simulink model "visualization_of_quad"  (R2015a)
settings: Solver=ode45  StartTime=0.0  StopTime=inf  RelTol=1e-3
values from neighbouring files (symbols this model uses):
  Beq = 0.2    [Parametres.m]
  Jeq = 0.005    [Parametres.m]
  Kb = 12    [Parametres.m]
  Kt = 12    [Parametres.m]
  Nl = 100    [Parametres.m]
  Nm = 200    [Parametres.m]
  Ra = 1100    [Parametres.m]
undefined symbols (not defined in the file or in its folder): sigbuilder_block
libraries: mblibv1 x34, simulink x5
settings Model: Creator=clien  LastModifiedBy=user
settings DataIOCC: SignalLoggingSaveFormat=ModelDataLogs
settings OptimizationCC: ExpressionDepthLimit=2147483647
settings DebuggingCC: UnderspecifiedInitializationDetection=Classic  MergeDetectMultiDrivingBlocksExec=none  SolverPrmCheckMsg=warning  FcnCallInpInsideContextMsg=UseLocalSettings  StateNameClashWarn=warning
settings GRTTargetCC: CombineOutputUpdateFcns=off  GRTInterface=on
settings SimMechanicsCC: VisOnUpdateDiagram=on  VisDuringSimulation=on  AutoFitVis=TIGHTFIT  LastVizWinPosition=[1 41 1366 627]  CamPosition=[6.82801;6.80801;6.82801;]  CamTarget=[-8.88178e-16;-0.02;-8.88178e-16;]  CamUpVector=[0;1;0;]  CamHeight=1.02417  VisBackgroundColor=[0.9;0.9;0.95;]  DefaultBodyColor=[1;0;0;]

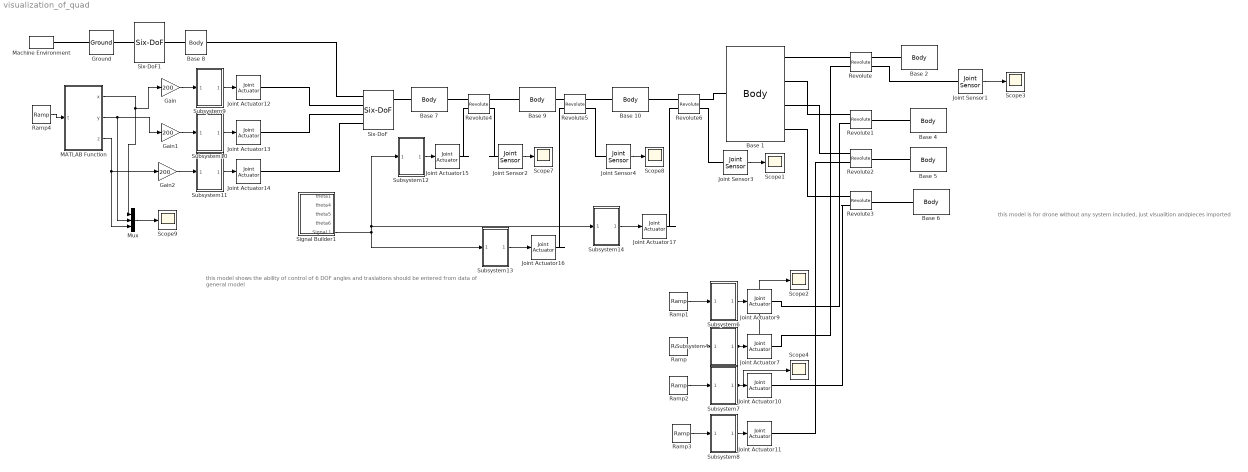
== system visualization_of_quad ==
  note: this model shows the ability of control of 6 DOF angles and traslations should be entered
      | from data of general model
  note: this model is for drone without any system included, just visualition andpieces imported
  Base 1 : mblibv1/Bodies/Body  LConnTagsString=CS1  RConnTagsString=CS5|CS4|CS3|CS2  UpdateFromCAD=off  DialogClass=MechanicalBodyBlock  Mass=.001  MassUnits=kg  InertiaUnits=kg*m^2  Inertia=eye(3)  Shape=Cylinder  ShapeDims=[1 1]  ShapeUnits=m  ShapeUse=false  Density=1  DensityUnits=kg/m^3  DensityUse=false  GraphicsMode=GFXFILE  GraphicsFileName=C:\Users\Oussama\Desktop\str file FINAL\framebody.stl  BodyColorSelMode=COLORPALETTE  BodyColor=[1 0.84314 0]  AttachedToCS=CS1  CG=Left$CG$[0 0 0]$World$CS1$mm$[0 0 0]$Euler X-Y-Z$deg$WORLD$false$none  WorkingFrames=Right$CS5$[0 30 -300]$Adjoining$CS1$mm$[0 0 0]$Euler X-Y-Z$deg$WORLD$true$none#Right$CS4$[0 30 300]$Adjoining$CS1$mm$[0 0 0]$Euler X-Y-Z$deg$WORLD$true$none#Right$CS3$[300 30 0]$Adjoining$CS1$mm$[0 0 0]$Euler X-Y-Z$deg$WORLD$true$none#Left$CS1$[0 0 0]$Adjoining$Adjoining$mm$[0 0 0]$Euler X-Y-Z$deg$WORLD$true$none#Right$CS2$[-300 30 0]$Adjoining$CS1$mm$[0 0 0]$Euler X-Y-Z$deg$WORLD$true$none  CGPos=[0 0 0]  CGRot=[0 0 0]  CS0Pos=[]  CS0Rot=[]  CS1Pos=[0 0 0]  CS1Rot=[0 0 0]  CS2Pos=[-300 30 0]  CS2Rot=[0 0 0]  CS3Pos=[300 30 0]  CS3Rot=[0 0 0]  CS4Pos=[0 30 300]  CS4Rot=[0 0 0]  CS5Pos=[0 30 -300]  CS5Rot=[0 0 0]  CS6Pos=[]  CS6Rot=[]  CS7Pos=[]  CS7Rot=[]  CS8Pos=[]  CS8Rot=[]  CS9Pos=[]  CS9Rot=[]  CS10Pos=[]  CS10Rot=[]  CS11Pos=[]  CS11Rot=[]  CS12Pos=[]  CS12Rot=[]  CS13Pos=[]  CS13Rot=[]  CS14Pos=[]  CS14Rot=[]  CS15Pos=[]  CS15Rot=[]  CS16Pos=[]  CS16Rot=[]  CS17Pos=[]  CS17Rot=[]  CS18Pos=[]  CS18Rot=[]  CS19Pos=[]  CS19Rot=[]  CS20Pos=[]  CS20Rot=[]
  Base 10 : mblibv1/Bodies/Body  LConnTagsString=CS1  RConnTagsString=CS2  UpdateFromCAD=off  DialogClass=MechanicalBodyBlock  Mass=0.00001  MassUnits=kg  InertiaUnits=kg*m^2  Inertia=eye(3)  Shape=Cylinder  ShapeDims=[1 1]  ShapeUnits=m  ShapeUse=false  Density=1  DensityUnits=kg/m^3  DensityUse=false  GraphicsMode=MACHINE_DEFAULT  GraphicsFileName=C:\Users\Oussama\Desktop\str file FINAL\framebody.stl  BodyColorSelMode=COLORPALETTE  BodyColor=[0 0 0]  AttachedToCS=CS1  CG=Left$CG$[0 0 0]$World$CS1$mm$[0 0 0]$Euler X-Y-Z$deg$WORLD$false$none  WorkingFrames=Left$CS1$[0 0 0]$Adjoining$Adjoining$mm$[0 0 0]$Euler X-Y-Z$deg$WORLD$true$none#Right$CS2$[0 0 0]$World$CS1$mm$[0 0 0]$Euler X-Y-Z$deg$WORLD$true$none  CGPos=[0 0 0]  CGRot=[0 0 0]  CS0Pos=[]  CS0Rot=[]  CS1Pos=[0 0 0]  CS1Rot=[0 0 0]  CS2Pos=[0 0 0]  CS2Rot=[0 0 0]  CS3Pos=[]  CS3Rot=[]  CS4Pos=[]  CS4Rot=[]  CS5Pos=[]  CS5Rot=[]  CS6Pos=[]  CS6Rot=[]  CS7Pos=[]  CS7Rot=[]  CS8Pos=[]  CS8Rot=[]  CS9Pos=[]  CS9Rot=[]  CS10Pos=[]  CS10Rot=[]  CS11Pos=[]  CS11Rot=[]  CS12Pos=[]  CS12Rot=[]  CS13Pos=[]  CS13Rot=[]  CS14Pos=[]  CS14Rot=[]  CS15Pos=[]  CS15Rot=[]  CS16Pos=[]  CS16Rot=[]  CS17Pos=[]  CS17Rot=[]  CS18Pos=[]  CS18Rot=[]  CS19Pos=[]  CS19Rot=[]  CS20Pos=[]  CS20Rot=[]
  Base 2 : mblibv1/Bodies/Body  LConnTagsString=CS1  RConnTagsString=CS2  UpdateFromCAD=off  DialogClass=MechanicalBodyBlock  Mass=0.000001  MassUnits=kg  InertiaUnits=kg*m^2  Inertia=eye(3)  Shape=Cylinder  ShapeDims=[1 1]  ShapeUnits=m  ShapeUse=false  Density=1  DensityUnits=kg/m^3  DensityUse=false  GraphicsMode=GFXFILE  GraphicsFileName=C:\Users\Oussama\Desktop\str file FINAL\proplers.stl  BodyColorSelMode=COLORPALETTE  BodyColor=[1 0 0]  AttachedToCS=CS1  CG=Left$CG$[0 0 0]$World$CS1$mm$[0 0 0]$Euler X-Y-Z$deg$WORLD$false$none  WorkingFrames=Left$CS1$[0 0 0]$Adjoining$Adjoining$mm$[0 0 0]$Euler X-Y-Z$deg$WORLD$true$none#Right$CS2$[0 0 0]$World$CS1$mm$[0 0 0]$Euler X-Y-Z$deg$WORLD$true$none  CGPos=[0 0 0]  CGRot=[0 0 0]  CS0Pos=[]  CS0Rot=[]  CS1Pos=[0 0 0]  CS1Rot=[0 0 0]  CS2Pos=[0 0 0]  CS2Rot=[0 0 0]  CS3Pos=[]  CS3Rot=[]  CS4Pos=[]  CS4Rot=[]  CS5Pos=[]  CS5Rot=[]  CS6Pos=[]  CS6Rot=[]  CS7Pos=[]  CS7Rot=[]  CS8Pos=[]  CS8Rot=[]  CS9Pos=[]  CS9Rot=[]  CS10Pos=[]  CS10Rot=[]  CS11Pos=[]  CS11Rot=[]  CS12Pos=[]  CS12Rot=[]  CS13Pos=[]  CS13Rot=[]  CS14Pos=[]  CS14Rot=[]  CS15Pos=[]  CS15Rot=[]  CS16Pos=[]  CS16Rot=[]  CS17Pos=[]  CS17Rot=[]  CS18Pos=[]  CS18Rot=[]  CS19Pos=[]  CS19Rot=[]  CS20Pos=[]  CS20Rot=[]
  Base 4 : mblibv1/Bodies/Body  LConnTagsString=CS1  RConnTagsString=CS2  UpdateFromCAD=off  DialogClass=MechanicalBodyBlock  Mass=0.000001  MassUnits=kg  InertiaUnits=kg*m^2  Inertia=eye(3)  Shape=Cylinder  ShapeDims=[1 1]  ShapeUnits=m  ShapeUse=false  Density=1  DensityUnits=kg/m^3  DensityUse=false  GraphicsMode=GFXFILE  GraphicsFileName=C:\Users\Oussama\Desktop\str file FINAL\proplers.stl  BodyColorSelMode=COLORPALETTE  BodyColor=[1 0 1]  AttachedToCS=CS1  CG=Left$CG$[0 0 0]$World$CS1$mm$[0 0 0]$Euler X-Y-Z$deg$WORLD$false$none  WorkingFrames=Left$CS1$[0 0 0]$Adjoining$Adjoining$mm$[0 0 0]$Euler X-Y-Z$deg$WORLD$true$none#Right$CS2$[0 0 0]$World$CS1$mm$[0 0 0]$Euler X-Y-Z$deg$WORLD$true$none  CGPos=[0 0 0]  CGRot=[0 0 0]  CS0Pos=[]  CS0Rot=[]  CS1Pos=[0 0 0]  CS1Rot=[0 0 0]  CS2Pos=[0 0 0]  CS2Rot=[0 0 0]  CS3Pos=[]  CS3Rot=[]  CS4Pos=[]  CS4Rot=[]  CS5Pos=[]  CS5Rot=[]  CS6Pos=[]  CS6Rot=[]  CS7Pos=[]  CS7Rot=[]  CS8Pos=[]  CS8Rot=[]  CS9Pos=[]  CS9Rot=[]  CS10Pos=[]  CS10Rot=[]  CS11Pos=[]  CS11Rot=[]  CS12Pos=[]  CS12Rot=[]  CS13Pos=[]  CS13Rot=[]  CS14Pos=[]  CS14Rot=[]  CS15Pos=[]  CS15Rot=[]  CS16Pos=[]  CS16Rot=[]  CS17Pos=[]  CS17Rot=[]  CS18Pos=[]  CS18Rot=[]  CS19Pos=[]  CS19Rot=[]  CS20Pos=[]  CS20Rot=[]
  Base 5 : mblibv1/Bodies/Body  LConnTagsString=CS1  RConnTagsString=CS2  UpdateFromCAD=off  DialogClass=MechanicalBodyBlock  Mass=0.000001  MassUnits=kg  InertiaUnits=kg*m^2  Inertia=eye(3)  Shape=Cylinder  ShapeDims=[1 1]  ShapeUnits=m  ShapeUse=false  Density=1  DensityUnits=kg/m^3  DensityUse=false  GraphicsMode=GFXFILE  GraphicsFileName=C:\Users\Oussama\Desktop\str file FINAL\proplers.stl  BodyColorSelMode=COLORPALETTE  BodyColor=[0 0 1]  AttachedToCS=CS1  CG=Left$CG$[0 0 0]$World$CS1$mm$[0 0 0]$Euler X-Y-Z$deg$WORLD$false$none  WorkingFrames=Left$CS1$[0 0 0]$Adjoining$Adjoining$mm$[0 0 0]$Euler X-Y-Z$deg$WORLD$true$none#Right$CS2$[0 0 0]$World$CS1$mm$[0 0 0]$Euler X-Y-Z$deg$WORLD$true$none  CGPos=[0 0 0]  CGRot=[0 0 0]  CS0Pos=[]  CS0Rot=[]  CS1Pos=[0 0 0]  CS1Rot=[0 0 0]  CS2Pos=[0 0 0]  CS2Rot=[0 0 0]  CS3Pos=[]  CS3Rot=[]  CS4Pos=[]  CS4Rot=[]  CS5Pos=[]  CS5Rot=[]  CS6Pos=[]  CS6Rot=[]  CS7Pos=[]  CS7Rot=[]  CS8Pos=[]  CS8Rot=[]  CS9Pos=[]  CS9Rot=[]  CS10Pos=[]  CS10Rot=[]  CS11Pos=[]  CS11Rot=[]  CS12Pos=[]  CS12Rot=[]  CS13Pos=[]  CS13Rot=[]  CS14Pos=[]  CS14Rot=[]  CS15Pos=[]  CS15Rot=[]  CS16Pos=[]  CS16Rot=[]  CS17Pos=[]  CS17Rot=[]  CS18Pos=[]  CS18Rot=[]  CS19Pos=[]  CS19Rot=[]  CS20Pos=[]  CS20Rot=[]
  Base 6 : mblibv1/Bodies/Body  LConnTagsString=CS1  RConnTagsString=CS2  UpdateFromCAD=off  DialogClass=MechanicalBodyBlock  Mass=0.000001  MassUnits=kg  InertiaUnits=kg*m^2  Inertia=eye(3)  Shape=Cylinder  ShapeDims=[1 1]  ShapeUnits=m  ShapeUse=false  Density=1  DensityUnits=kg/m^3  DensityUse=false  GraphicsMode=GFXFILE  GraphicsFileName=C:\Users\Oussama\Desktop\str file FINAL\proplers.stl  BodyColorSelMode=COLORPALETTE  BodyColor=[0 1 0]  AttachedToCS=CS1  CG=Left$CG$[0 0 0]$World$CS1$mm$[0 0 0]$Euler X-Y-Z$deg$WORLD$false$none  WorkingFrames=Left$CS1$[0 0 0]$Adjoining$Adjoining$mm$[0 0 0]$Euler X-Y-Z$deg$WORLD$true$none#Right$CS2$[0 0 0]$World$CS1$mm$[0 0 0]$Euler X-Y-Z$deg$WORLD$true$none  CGPos=[0 0 0]  CGRot=[0 0 0]  CS0Pos=[]  CS0Rot=[]  CS1Pos=[0 0 0]  CS1Rot=[0 0 0]  CS2Pos=[0 0 0]  CS2Rot=[0 0 0]  CS3Pos=[]  CS3Rot=[]  CS4Pos=[]  CS4Rot=[]  CS5Pos=[]  CS5Rot=[]  CS6Pos=[]  CS6Rot=[]  CS7Pos=[]  CS7Rot=[]  CS8Pos=[]  CS8Rot=[]  CS9Pos=[]  CS9Rot=[]  CS10Pos=[]  CS10Rot=[]  CS11Pos=[]  CS11Rot=[]  CS12Pos=[]  CS12Rot=[]  CS13Pos=[]  CS13Rot=[]  CS14Pos=[]  CS14Rot=[]  CS15Pos=[]  CS15Rot=[]  CS16Pos=[]  CS16Rot=[]  CS17Pos=[]  CS17Rot=[]  CS18Pos=[]  CS18Rot=[]  CS19Pos=[]  CS19Rot=[]  CS20Pos=[]  CS20Rot=[]
  Base 7 : mblibv1/Bodies/Body  LConnTagsString=CS1  RConnTagsString=CS2  UpdateFromCAD=off  DialogClass=MechanicalBodyBlock  Mass=100000  MassUnits=kg  InertiaUnits=kg*m^2  Inertia=1000000*eye(3)  Shape=Cylinder  ShapeDims=[1 1]  ShapeUnits=m  ShapeUse=false  Density=1  DensityUnits=kg/m^3  DensityUse=false  GraphicsMode=MACHINE_DEFAULT  GraphicsFileName=C:\Users\Oussama\Desktop\str file FINAL\framebody.stl  BodyColorSelMode=COLORPALETTE  BodyColor=[0 0 0]  AttachedToCS=CS1  CG=Left$CG$[0 0 0]$World$CS1$mm$[0 0 0]$Euler X-Y-Z$deg$WORLD$false$none  WorkingFrames=Left$CS1$[0 0 0]$Adjoining$Adjoining$mm$[0 0 0]$Euler X-Y-Z$deg$WORLD$true$none#Right$CS2$[0 0 0]$World$CS1$mm$[0 0 0]$Euler X-Y-Z$deg$WORLD$true$none  CGPos=[0 0 0]  CGRot=[0 0 0]  CS0Pos=[]  CS0Rot=[]  CS1Pos=[0 0 0]  CS1Rot=[0 0 0]  CS2Pos=[0 0 0]  CS2Rot=[0 0 0]  CS3Pos=[]  CS3Rot=[]  CS4Pos=[]  CS4Rot=[]  CS5Pos=[]  CS5Rot=[]  CS6Pos=[]  CS6Rot=[]  CS7Pos=[]  CS7Rot=[]  CS8Pos=[]  CS8Rot=[]  CS9Pos=[]  CS9Rot=[]  CS10Pos=[]  CS10Rot=[]  CS11Pos=[]  CS11Rot=[]  CS12Pos=[]  CS12Rot=[]  CS13Pos=[]  CS13Rot=[]  CS14Pos=[]  CS14Rot=[]  CS15Pos=[]  CS15Rot=[]  CS16Pos=[]  CS16Rot=[]  CS17Pos=[]  CS17Rot=[]  CS18Pos=[]  CS18Rot=[]  CS19Pos=[]  CS19Rot=[]  CS20Pos=[]  CS20Rot=[]
  Base 8 : mblibv1/Bodies/Body  LConnTagsString=CS1  RConnTagsString=CS2  UpdateFromCAD=off  DialogClass=MechanicalBodyBlock  Mass=100000000000000000000  MassUnits=kg  InertiaUnits=kg*m^2  Inertia=10000000000000000*eye(3)  Shape=Cylinder  ShapeDims=[1 1]  ShapeUnits=m  ShapeUse=false  Density=1  DensityUnits=kg/m^3  DensityUse=false  GraphicsMode=MACHINE_DEFAULT  GraphicsFileName=C:\Users\Oussama\Desktop\str file FINAL\framebody.stl  BodyColorSelMode=COLORPALETTE  BodyColor=[0 0 0]  AttachedToCS=CS1  CG=Left$CG$[0 0 0]$World$CS1$mm$[0 0 0]$Euler X-Y-Z$deg$WORLD$false$none  WorkingFrames=Left$CS1$[0 0 0]$Adjoining$Adjoining$mm$[0 0 0]$Euler X-Y-Z$deg$WORLD$true$none#Right$CS2$[0 0 0]$World$CS1$mm$[0 0 0]$Euler X-Y-Z$deg$WORLD$true$none  CGPos=[0 0 0]  CGRot=[0 0 0]  CS0Pos=[]  CS0Rot=[]  CS1Pos=[0 0 0]  CS1Rot=[0 0 0]  CS2Pos=[0 0 0]  CS2Rot=[0 0 0]  CS3Pos=[]  CS3Rot=[]  CS4Pos=[]  CS4Rot=[]  CS5Pos=[]  CS5Rot=[]  CS6Pos=[]  CS6Rot=[]  CS7Pos=[]  CS7Rot=[]  CS8Pos=[]  CS8Rot=[]  CS9Pos=[]  CS9Rot=[]  CS10Pos=[]  CS10Rot=[]  CS11Pos=[]  CS11Rot=[]  CS12Pos=[]  CS12Rot=[]  CS13Pos=[]  CS13Rot=[]  CS14Pos=[]  CS14Rot=[]  CS15Pos=[]  CS15Rot=[]  CS16Pos=[]  CS16Rot=[]  CS17Pos=[]  CS17Rot=[]  CS18Pos=[]  CS18Rot=[]  CS19Pos=[]  CS19Rot=[]  CS20Pos=[]  CS20Rot=[]
  Base 9 : mblibv1/Bodies/Body  LConnTagsString=CS1  RConnTagsString=CS2  UpdateFromCAD=off  DialogClass=MechanicalBodyBlock  Mass=0.00001  MassUnits=kg  InertiaUnits=kg*m^2  Inertia=eye(3)  Shape=Cylinder  ShapeDims=[1 1]  ShapeUnits=m  ShapeUse=false  Density=1  DensityUnits=kg/m^3  DensityUse=false  GraphicsMode=MACHINE_DEFAULT  GraphicsFileName=C:\Users\Oussama\Desktop\str file FINAL\framebody.stl  BodyColorSelMode=COLORPALETTE  BodyColor=[0 0 0]  AttachedToCS=CS1  CG=Left$CG$[0 0 0]$World$CS1$mm$[0 0 0]$Euler X-Y-Z$deg$WORLD$false$none  WorkingFrames=Left$CS1$[0 0 0]$Adjoining$Adjoining$mm$[0 0 0]$Euler X-Y-Z$deg$WORLD$true$none#Right$CS2$[0 0 0]$World$CS1$mm$[0 0 0]$Euler X-Y-Z$deg$WORLD$true$none  CGPos=[0 0 0]  CGRot=[0 0 0]  CS0Pos=[]  CS0Rot=[]  CS1Pos=[0 0 0]  CS1Rot=[0 0 0]  CS2Pos=[0 0 0]  CS2Rot=[0 0 0]  CS3Pos=[]  CS3Rot=[]  CS4Pos=[]  CS4Rot=[]  CS5Pos=[]  CS5Rot=[]  CS6Pos=[]  CS6Rot=[]  CS7Pos=[]  CS7Rot=[]  CS8Pos=[]  CS8Rot=[]  CS9Pos=[]  CS9Rot=[]  CS10Pos=[]  CS10Rot=[]  CS11Pos=[]  CS11Rot=[]  CS12Pos=[]  CS12Rot=[]  CS13Pos=[]  CS13Rot=[]  CS14Pos=[]  CS14Rot=[]  CS15Pos=[]  CS15Rot=[]  CS16Pos=[]  CS16Rot=[]  CS17Pos=[]  CS17Rot=[]  CS18Pos=[]  CS18Rot=[]  CS19Pos=[]  CS19Rot=[]  CS20Pos=[]  CS20Rot=[]
  Gain : Gain  Gain=200
  Gain1 : Gain  Gain=200
  Gain2 : Gain  Gain=200
  Ground : mblibv1/Bodies/Ground  UpdateFromCAD=off  LeftPortType=env  RightPortType=workingframe  PhysicalDomain=Mechanical  DialogClass=GroundBlock  CoordPosition=[0 0 0]  CoordPositionUnits=m  StateVectorMgrId=0  MachineId=[1 0]  ShowEnvPort=on  ParameterChecksum=[2469406994, 1823206531, 3009068099, 3398779523]  TopologyChecksum=[157137947, 283279318, 358089753, 4107751040]
  Joint Actuator10 : mblibv1/Sensors &  Actuators/Joint Actuator  UpdateFromCAD=off  PhysicalDomain=Mechanical  PortType=blob  ActuationStyle=Motion  AngleUnits=rev  ArcVelocityUnits=rpm  ArcAccelerationUnits=rad/s^2  CoordPositionUnits=m  VelocityUnits=m/s  AccelerationUnits=m/s^2  ForceUnits=N  TorqueUnits=N*m  ActiveIO=on  Width=3  DialogClass=MechanicalActuatorBlock  Primitive=R1  ReferenceFrame=Absolute (World)
  Joint Actuator11 : mblibv1/Sensors &  Actuators/Joint Actuator  UpdateFromCAD=off  PhysicalDomain=Mechanical  PortType=blob  ActuationStyle=Motion  AngleUnits=rev  ArcVelocityUnits=rad/s  ArcAccelerationUnits=rad/s^2  CoordPositionUnits=m  VelocityUnits=m/s  AccelerationUnits=m/s^2  ForceUnits=N  TorqueUnits=N*m  ActiveIO=on  Width=3  DialogClass=MechanicalActuatorBlock  Primitive=R1  ReferenceFrame=Absolute (World)
  Joint Actuator12 : mblibv1/Sensors &  Actuators/Joint Actuator  UpdateFromCAD=off  PhysicalDomain=Mechanical  PortType=blob  ActuationStyle=Motion  AngleUnits=rev  ArcVelocityUnits=rpm  ArcAccelerationUnits=rad/s^2  CoordPositionUnits=mm  VelocityUnits=m/s  AccelerationUnits=m/s^2  ForceUnits=N  TorqueUnits=N*m  ActiveIO=on  Width=3  DialogClass=MechanicalActuatorBlock  Primitive=P1  ReferenceFrame=Absolute (World)
  Joint Actuator13 : mblibv1/Sensors &  Actuators/Joint Actuator  UpdateFromCAD=off  PhysicalDomain=Mechanical  PortType=blob  ActuationStyle=Motion  AngleUnits=rev  ArcVelocityUnits=rpm  ArcAccelerationUnits=rad/s^2  CoordPositionUnits=mm  VelocityUnits=m/s  AccelerationUnits=m/s^2  ForceUnits=N  TorqueUnits=N*m  ActiveIO=on  Width=3  DialogClass=MechanicalActuatorBlock  Primitive=P3  ReferenceFrame=Absolute (World)
  Joint Actuator14 : mblibv1/Sensors &  Actuators/Joint Actuator  UpdateFromCAD=off  PhysicalDomain=Mechanical  PortType=blob  ActuationStyle=Motion  AngleUnits=rev  ArcVelocityUnits=rpm  ArcAccelerationUnits=rad/s^2  CoordPositionUnits=mm  VelocityUnits=m/s  AccelerationUnits=m/s^2  ForceUnits=N  TorqueUnits=N*m  ActiveIO=on  Width=3  DialogClass=MechanicalActuatorBlock  Primitive=P2  ReferenceFrame=Absolute (World)
  Joint Actuator15 : mblibv1/Sensors &  Actuators/Joint Actuator  UpdateFromCAD=off  PhysicalDomain=Mechanical  PortType=blob  ActuationStyle=Motion  AngleUnits=deg  ArcVelocityUnits=deg/s  ArcAccelerationUnits=deg/s^2  CoordPositionUnits=mm  VelocityUnits=m/s  AccelerationUnits=m/s^2  ForceUnits=N  TorqueUnits=N*m  ActiveIO=on  Width=3  DialogClass=MechanicalActuatorBlock  Primitive=R1  ReferenceFrame=Absolute (World)
  Joint Actuator16 : mblibv1/Sensors &  Actuators/Joint Actuator  UpdateFromCAD=off  PhysicalDomain=Mechanical  PortType=blob  ActuationStyle=Motion  AngleUnits=deg  ArcVelocityUnits=deg/s  ArcAccelerationUnits=deg/s^2  CoordPositionUnits=mm  VelocityUnits=m/s  AccelerationUnits=m/s^2  ForceUnits=N  TorqueUnits=N*m  ActiveIO=on  Width=3  DialogClass=MechanicalActuatorBlock  Primitive=R1  ReferenceFrame=Absolute (World)
  Joint Actuator17 : mblibv1/Sensors &  Actuators/Joint Actuator  UpdateFromCAD=off  PhysicalDomain=Mechanical  PortType=blob  ActuationStyle=Motion  AngleUnits=deg  ArcVelocityUnits=deg/s  ArcAccelerationUnits=deg/s^2  CoordPositionUnits=mm  VelocityUnits=m/s  AccelerationUnits=m/s^2  ForceUnits=N  TorqueUnits=N*m  ActiveIO=on  Width=3  DialogClass=MechanicalActuatorBlock  Primitive=R1  ReferenceFrame=Absolute (World)
  Joint Actuator7 : mblibv1/Sensors &  Actuators/Joint Actuator  UpdateFromCAD=off  PhysicalDomain=Mechanical  PortType=blob  ActuationStyle=Motion  AngleUnits=rev  ArcVelocityUnits=rpm  ArcAccelerationUnits=rad/s^2  CoordPositionUnits=m  VelocityUnits=m/s  AccelerationUnits=m/s^2  ForceUnits=N  TorqueUnits=N*m  ActiveIO=on  Width=3  DialogClass=MechanicalActuatorBlock  Primitive=R1  ReferenceFrame=Absolute (World)
  Joint Actuator9 : mblibv1/Sensors &  Actuators/Joint Actuator  UpdateFromCAD=off  PhysicalDomain=Mechanical  PortType=blob  ActuationStyle=Motion  AngleUnits=rev  ArcVelocityUnits=rpm  ArcAccelerationUnits=rad/s^2  CoordPositionUnits=m  VelocityUnits=m/s  AccelerationUnits=m/s^2  ForceUnits=N  TorqueUnits=N*m  ActiveIO=on  Width=3  DialogClass=MechanicalActuatorBlock  Primitive=R1  ReferenceFrame=Absolute (World)
  Joint Sensor1 : mblibv1/Sensors &  Actuators/Joint Sensor  UpdateFromCAD=off  PhysicalDomain=Mechanical  PortType=blob  Muxed=on  Pose=off  Angle=on  AngleUnits=deg  ArcVelocity=off  ArcVelocityUnits=deg/s  ArcAcceleration=off  ArcAccelerationUnits=deg/s^2  CoordPosition=on  CoordPositionUnits=m  Velocity=on  VelocityUnits=m/s  Acceleration=off  AccelerationUnits=m/s^2  Quaternion=on  QuaternionDT=on  QuaternionDDT=on  QuaternionUnits=off  OutputVector=[1]  ActiveIO=on  Width=1  DialogClass=MechanicalSensorBlock  Primitive=R1  Force=off  ForceUnits=N  Torque=off  TorqueUnits=N*m  ReferenceFrame=Absolute (World)  ReactionSensedSide=Base  ReactionReferenceFrame=Absolute (World)  ReactionForce=off  ReactionForceUnits=N  ReactionMoment=off  ReactionMomentUnits=N*m
  Joint Sensor2 : mblibv1/Sensors &  Actuators/Joint Sensor  UpdateFromCAD=off  PhysicalDomain=Mechanical  PortType=blob  Muxed=on  Pose=off  Angle=on  AngleUnits=deg  ArcVelocity=on  ArcVelocityUnits=deg/s  ArcAcceleration=on  ArcAccelerationUnits=deg/s^2  CoordPosition=on  CoordPositionUnits=m  Velocity=off  VelocityUnits=m/s  Acceleration=off  AccelerationUnits=m/s^2  Quaternion=on  QuaternionDT=off  QuaternionDDT=off  QuaternionUnits=off  OutputVector=[1]  ActiveIO=on  Width=3  DialogClass=MechanicalSensorBlock  Primitive=R1  Force=off  ForceUnits=N  Torque=off  TorqueUnits=N*m  ReferenceFrame=Absolute (World)  ReactionSensedSide=Base  ReactionReferenceFrame=Absolute (World)  ReactionForce=off  ReactionForceUnits=N  ReactionMoment=off  ReactionMomentUnits=N*m
  Joint Sensor3 : mblibv1/Sensors &  Actuators/Joint Sensor  UpdateFromCAD=off  PhysicalDomain=Mechanical  PortType=blob  Muxed=on  Pose=off  Angle=on  AngleUnits=deg  ArcVelocity=on  ArcVelocityUnits=deg/s  ArcAcceleration=on  ArcAccelerationUnits=deg/s^2  CoordPosition=on  CoordPositionUnits=m  Velocity=off  VelocityUnits=m/s  Acceleration=off  AccelerationUnits=m/s^2  Quaternion=on  QuaternionDT=off  QuaternionDDT=off  QuaternionUnits=off  OutputVector=[1]  ActiveIO=on  Width=3  DialogClass=MechanicalSensorBlock  Primitive=R1  Force=off  ForceUnits=N  Torque=off  TorqueUnits=N*m  ReferenceFrame=Absolute (World)  ReactionSensedSide=Base  ReactionReferenceFrame=Absolute (World)  ReactionForce=off  ReactionForceUnits=N  ReactionMoment=off  ReactionMomentUnits=N*m
  Joint Sensor4 : mblibv1/Sensors &  Actuators/Joint Sensor  UpdateFromCAD=off  PhysicalDomain=Mechanical  PortType=blob  Muxed=on  Pose=off  Angle=on  AngleUnits=deg  ArcVelocity=on  ArcVelocityUnits=deg/s  ArcAcceleration=on  ArcAccelerationUnits=deg/s^2  CoordPosition=on  CoordPositionUnits=m  Velocity=off  VelocityUnits=m/s  Acceleration=off  AccelerationUnits=m/s^2  Quaternion=on  QuaternionDT=off  QuaternionDDT=off  QuaternionUnits=off  OutputVector=[1]  ActiveIO=on  Width=3  DialogClass=MechanicalSensorBlock  Primitive=R1  Force=off  ForceUnits=N  Torque=off  TorqueUnits=N*m  ReferenceFrame=Absolute (World)  ReactionSensedSide=Base  ReactionReferenceFrame=Absolute (World)  ReactionForce=off  ReactionForceUnits=N  ReactionMoment=off  ReactionMomentUnits=N*m
  MATLAB Function : MATLAB Function  TreatAsAtomicUnit=on
  Machine Environment : mblibv1/Bodies/Machine Environment  PortType=env  PhysicalDomain=Mechanical  DialogTemplateClass=MECH.MachineEnvironment  SyncWhenCopied=off  Gravity=[0 0. 0]  GravityUnits=m/s^2  GravityAsSignal=off  Dimensionality=Auto-detect  AnalysisType=Forward dynamics  LinearAssemblyTolerance=1  LinearAssemblyToleranceUnits=m  AngularAssemblyTolerance=1e-3  AngularAssemblyToleranceUnits=rad  ConstraintSolverType=Stabilizing  ConstraintRelTolerance=1e-4  ConstraintAbsTolerance=1e-4  UseRobustSingularityHandling=off  RedundancyAnalysisToleranceType=Automatically select tolerance  RedundancyAnalysisTolerance=1e-14  StatePerturbationType=Fixed  PerturbationSize=1e-5  VisualizeMachine=on  BodyVisualizationType=Use model default body geometries  BodyColorSelMode=Use model default  DefaultBodyColor=[1 0 0]
  Mux : Mux  Inputs=3
  Ramp : simulink/Sources/Ramp  slope=8000  start=0  X0=0
  Ramp1 : simulink/Sources/Ramp  slope=8000  start=0  X0=0
  Ramp2 : simulink/Sources/Ramp  slope=-8000  start=0  X0=0
  Ramp3 : simulink/Sources/Ramp  slope=-8000  start=0  X0=0
  Ramp4 : simulink/Sources/Ramp  slope=1  start=0  X0=0
  Revolute : mblibv1/Joints/Revolute  LConnTagsString=__newl0|SA1  RConnTagsString=__newr0|SA1  UpdateFromCAD=off  NumSAPorts=2  CutJoint=off  MarkAsCut=off  Primitives=prismatic  PrimitiveProps=R1$World$[0 1 0]$revolute  DialogClass=JointBlock  R1Axis=[0 1 0]
  Revolute1 : mblibv1/Joints/Revolute  LConnTagsString=__newl0|SA1  RConnTagsString=__newr0  UpdateFromCAD=off  NumSAPorts=1  CutJoint=off  MarkAsCut=off  Primitives=prismatic  PrimitiveProps=R1$World$[0 1 0]$revolute  DialogClass=JointBlock  R1Axis=[0 1 0]
  Revolute2 : mblibv1/Joints/Revolute  LConnTagsString=__newl0|SA1  RConnTagsString=__newr0  UpdateFromCAD=off  NumSAPorts=1  CutJoint=off  MarkAsCut=off  Primitives=prismatic  PrimitiveProps="R1$World$[0  1 0]$revolute"  DialogClass=JointBlock  R1Axis="[0  1 0]"
  Revolute3 : mblibv1/Joints/Revolute  LConnTagsString=__newl0|SA1  RConnTagsString=__newr0  UpdateFromCAD=off  NumSAPorts=1  CutJoint=off  MarkAsCut=off  Primitives=prismatic  PrimitiveProps=R1$World$[0 1 0]$revolute  DialogClass=JointBlock  R1Axis=[0 1 0]
  Revolute4 : mblibv1/Joints/Revolute  LConnTagsString=__newl0|SA1  RConnTagsString=__newr0|SA1  UpdateFromCAD=off  NumSAPorts=2  CutJoint=off  MarkAsCut=off  Primitives=prismatic  PrimitiveProps=R1$World$[0 1 0]$revolute  DialogClass=JointBlock  R1Axis=[0 1 0]
  Revolute5 : mblibv1/Joints/Revolute  LConnTagsString=__newl0|SA1  RConnTagsString=__newr0|SA1  UpdateFromCAD=off  NumSAPorts=2  CutJoint=off  MarkAsCut=off  Primitives=prismatic  PrimitiveProps=R1$World$[1 0 0]$revolute  DialogClass=JointBlock  R1Axis=[1 0 0]
  Revolute6 : mblibv1/Joints/Revolute  LConnTagsString=__newl0|SA1  RConnTagsString=__newr0|SA1  UpdateFromCAD=off  NumSAPorts=2  CutJoint=off  MarkAsCut=off  Primitives=prismatic  PrimitiveProps=R1$World$[0 0 1]$revolute  DialogClass=JointBlock  R1Axis=[0 0 1]
  Scope{1..4,7..9} (7 alike) : Scope
      Scope1 settings: YMin=89.997  YMax=90.003
      Scope2 settings: YMin=1  YMax=7  SaveName=ScopeData2
      Scope3 settings: YMin=-200  YMax=200  SaveName=ScopeData3
      Scope4 settings: YMin=1  YMax=7  SaveName=ScopeData4
      Scope7 settings: YMin=89.997  YMax=90.003  SaveName=ScopeData8
      Scope8 settings: YMin=89.997  YMax=90.003  SaveName=ScopeData9
      Scope9 settings: YMin=-7.5  YMax=10  SaveName=ScopeData10
  Signal Builder1 : Subsystem  Tag=STV Subsys  LoadFcn=sigbuilder_block('load');  StartFcn=sigbuilder_block('start');  StopFcn=sigbuilder_block('stop');  ClipboardFcn=sigbuilder_block('clipboard');  mask(Sigbuilder block){}
      mask help: Create and generate interchangeable groups of signals whose waveforms are piecewise linear.
      mask init:
      | if ~strcmp(get_param(bdroot(gcbh),'SimulationStatus'),'stopped') tuvar = sigbuilder_block('maskInit'); end
      settings: CopyFcn=sigbuilder_block('copy');  DeleteFcn=sigbuilder_block('delete');  ModelCloseFcn=sigbuilder_block('modelClose');  PreSaveFcn=sigbuilder_block('preSave');  PauseFcn=sigbuilder_block('pause')  ContinueFcn=sigbuilder_block('continue')  NameChangeFcn=sigbuilder_block('namechange');  OpenFcn=sigbuilder_block('open',[214.5 69 550.5 394.5 ]);  CloseFcn=sigbuilder_block('close');
      mask Display: plot(0, 0, 100, 100,[2, 2, 32, 32, 2], [68, 8, 8, 68, 68],[32, 2], [38, 38], [32, 19, 2],[53, 60, 44], [32, 17, 17, 2],[16, 16, 31, 31]);txt = getActiveGroup(gcbh);text(2, 100, txt,'verticalAlignment', 'top');
  Six-DoF : mblibv1/Joints/Six-DoF  LConnTagsString=__newl0|SA1|SA2|SA3  RConnTagsString=__newr0|SA1|SA2  UpdateFromCAD=off  NumSAPorts=5  CutJoint=off  MarkAsCut=off  Primitives=prismatic_prismatic  PrimitiveProps=P1$World$[1 0 0]$prismatic#P2$World$[0 1 0]$prismatic#P3$World$[0 0 1]$prismatic#S$World$[0 0 0]$spherical  DialogClass=JointBlock  P1Axis=[1 0 0]  P2Axis=[0 1 0]  P3Axis=[0 0 1]  SAxis=[0 0 0]
  Six-DoF1 : mblibv1/Joints/Six-DoF  LConnTagsString=__newl0  RConnTagsString=__newr0  UpdateFromCAD=off  NumSAPorts=0  CutJoint=off  MarkAsCut=off  Primitives=prismatic_prismatic  PrimitiveProps=P1$World$[1 0 0]$prismatic#P2$World$[0 1 0]$prismatic#P3$World$[0 0 1]$prismatic#S$World$[0 0 0]$spherical  DialogClass=JointBlock  P1Axis=[1 0 0]  P2Axis=[0 1 0]  P3Axis=[0 0 1]  SAxis=[0 0 0]
  Subsystem10 : Subsystem
  Subsystem11 : Subsystem
  Subsystem12 : Subsystem
  Subsystem13 : Subsystem
  Subsystem14 : Subsystem
  Subsystem4 : Subsystem
  Subsystem6 : Subsystem
  Subsystem7 : Subsystem
  Subsystem8 : Subsystem
  Subsystem9 : Subsystem
  wires:
  Ramp/1 -> Subsystem4/1(In1)
  Subsystem6/1(Out1) -> Joint Actuator9/1
  Ramp1/1 -> Subsystem6/1(In1)
  Subsystem7/1(Out1) -> Scope4/1, Joint Actuator10/1
  Ramp2/1 -> Subsystem7/1(In1)
  Subsystem8/1(Out1) -> Joint Actuator11/1
  Ramp3/1 -> Subsystem8/1(In1)
  Joint Sensor1/1 -> Scope3/1
  Subsystem4/1(Out1) -> Scope2/1, Joint Actuator7/1
  Subsystem9/1(Out1) -> Joint Actuator12/1
  Subsystem10/1(Out1) -> Joint Actuator13/1
  Subsystem11/1(Out1) -> Joint Actuator14/1
  Subsystem12/1(Out1) -> Joint Actuator15/1
  Joint Sensor2/1 -> Scope7/1
  Subsystem13/1(Out1) -> Joint Actuator16/1
  Joint Sensor4/1 -> Scope8/1
  Subsystem14/1(Out1) -> Joint Actuator17/1
  Signal Builder1/5(Signal 1) -> Subsystem13/1(In1), Subsystem14/1(In1), Subsystem12/1(In1)
  Ramp4/1 -> MATLAB Function/1(t)
  MATLAB Function/1(x) -> Gain/1, Mux/1
  MATLAB Function/2(y) -> Mux/2, Gain1/1
  MATLAB Function/3(z) -> Mux/3, Gain2/1
  Mux/1 -> Scope9/1
  Gain/1 -> Subsystem9/1(In1)
  Gain1/1 -> Subsystem10/1(In1)
  Gain2/1 -> Subsystem11/1(In1)
  Joint Sensor3/1 -> Scope1/1
  connections:
  Ground/LConn1 -- Machine Environment/RConn1
  Six-DoF1/LConn1 -- Ground/RConn1
  Revolute/RConn1 -- Base 2/LConn1
  Revolute/LConn1 -- Base 1/RConn1
  Base 6/LConn1 -- Revolute3/RConn1
  Revolute3/LConn1 -- Base 1/RConn4
  Base 5/LConn1 -- Revolute2/RConn1
  Revolute2/LConn1 -- Base 1/RConn3
  Base 4/LConn1 -- Revolute1/RConn1
  Revolute1/LConn1 -- Base 1/RConn2
  Joint Actuator7/RConn1 -- Revolute/LConn2
  Revolute1/LConn2 -- Joint Actuator9/RConn1
  Revolute3/LConn2 -- Joint Actuator10/RConn1
  Joint Actuator11/RConn1 -- Revolute2/LConn2
  Joint Sensor1/LConn1 -- Revolute/RConn2
  Joint Actuator12/RConn1 -- Six-DoF/LConn2
  Joint Actuator13/RConn1 -- Six-DoF/LConn3
  Joint Actuator14/RConn1 -- Six-DoF/LConn4
  Base 7/LConn1 -- Six-DoF/RConn1
  Revolute4/LConn1 -- Base 7/RConn1
  Joint Actuator15/RConn1 -- Revolute4/LConn2
  Joint Sensor2/LConn1 -- Revolute4/RConn2
  Base 8/LConn1 -- Six-DoF1/RConn1
  Six-DoF/LConn1 -- Base 8/RConn1
  Joint Actuator16/RConn1 -- Revolute5/LConn2
  Revolute5/RConn2 -- Joint Sensor4/LConn1
  Revolute5/LConn1 -- Base 9/RConn1
  Revolute6/LConn1 -- Base 10/RConn1
  Base 9/LConn1 -- Revolute4/RConn1
  Revolute5/RConn1 -- Base 10/LConn1
  Revolute6/RConn1 -- Base 1/LConn1
  Joint Actuator17/RConn1 -- Revolute6/LConn2
  Joint Sensor3/LConn1 -- Revolute6/RConn2

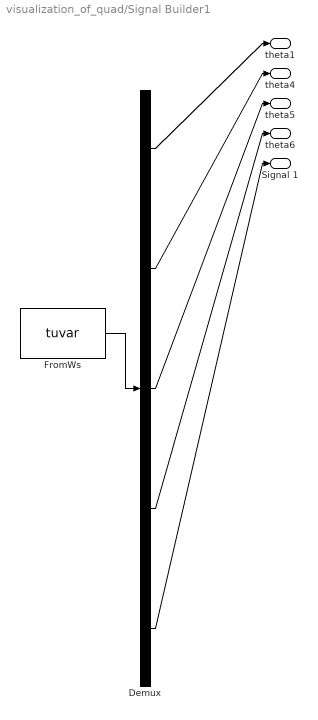
== system visualization_of_quad/Signal Builder1 ==
  Demux : Demux  Tag=STV Demux  Outputs=5
  FromWs : FromWorkspace  Tag=STV FromWs  VariableName=tuvar  SampleTime=0
      SigBuilderData=|
      | common.afterFinalStr = 'Extrapolate'
      | common.sampleTime = 0
      | dataSet.timeRange = [0 100]
      | dataSet.name = 'Group 1'
      | sbobj.Groups.Name = 'Group 1'
      | sbobj.Groups.Signals(1).Name = 'theta1'
      | sbobj.Groups.Signals(1).XData = [0 0.8 0.8 3 3 100]
      | sbobj.Groups.Signals(1).YData = [0 0 -6 -6 0 0]
      | sbobj.Groups.Signals(2).Name = 'theta4'
      | sbobj.Groups.Signals(2).XData = [0 4.8 4.8 6.3 7.8 7.8 100]
      | sbobj.Groups.Signals(2).YData = [0 0 -90 -90 -90 0 0]
      | sbobj.Groups.Signals(3).Name = 'theta5'
      | sbobj.Groups.Signals(3).XData = [0 9.6 9.6 12 12 14.2 14.2 100]
      | sbobj.Groups.Signals(3).YData = [0 0 180 180 -180 -180 0 0]
      | sbobj.Groups.Signals(4).Name = 'theta6'
      | sbobj.Groups.Signals(4).XData = [0 12.1 12.1 13.6 13.6 15.1 15.1 100]
      | sbobj.Groups.Signals(4).YData = [0 0 90 90 -90 -90 0 0]
      | sbobj.Groups.Signals(5).Name = 'Signal 1'
      | sbobj.Groups.Signals(5).XData = [0 40 60 100]
      | sbobj.Groups.Signals(5).YData = [0 0 0 0]
      | sbobj.Groups.TimeRange = [0 100]
  theta1 : Outport  Tag=STV Outport
  theta4 : Outport  Tag=STV Outport  Port=2
  theta5 : Outport  Tag=STV Outport  Port=3
  theta6 : Outport  Tag=STV Outport  Port=4
  Signal 1 : Outport  Tag=STV Outport  Port=5
  wires:
  FromWs/1 -> Demux/1
  Demux/1 -> theta1/1
  Demux/2 -> theta4/1
  Demux/3 -> theta5/1
  Demux/4 -> theta6/1
  Demux/5 -> Signal 1/1

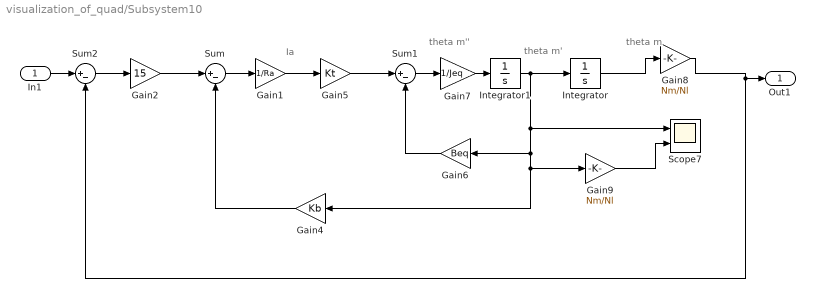
== system visualization_of_quad/Subsystem10 ==
  note: theta m''
  note: theta m'
  note: theta m
  note: Ia
  In1 : Inport
  Gain1 : Gain  Gain=1/Ra
  Gain2 : Gain  Gain=15
  Gain4 : Gain  Gain=Kb
  Gain5 : Gain  Gain=Kt
  Gain6 : Gain  Gain=Beq
  Gain7 : Gain  Gain=1/Jeq
  Gain8 : Gain  Gain=Nm/Nl
  Gain9 : Gain  Gain=Nm/Nl
  Integrator : Integrator
  Integrator1 : Integrator
  Scope7 : Scope  NumInputPorts=2
      settings: YMin=5.04527e-12~1.26132e-12  YMax=5.04527e-12~1.26132e-12  SaveName=ScopeData7
  Sum : Sum  Inputs=|+-
  Sum1 : Sum  Inputs=|+-
  Sum2 : Sum  Inputs=|+-
  Out1 : Outport
  wires:
  Sum/1 -> Gain1/1
  Gain4/1 -> Sum/2
  Integrator1/1 -> Gain9/1, Gain4/1, Gain6/1, Scope7/1, Integrator/1
  Gain1/1 -> Gain5/1
  Gain5/1 -> Sum1/1
  Gain6/1 -> Sum1/2
  Sum1/1 -> Gain7/1
  Gain7/1 -> Integrator1/1
  Integrator/1 -> Gain8/1
  Gain8/1 -> Sum2/2, Out1/1
  Gain9/1 -> Scope7/2
  Sum2/1 -> Gain2/1
  In1/1 -> Sum2/1
  Gain2/1 -> Sum/1

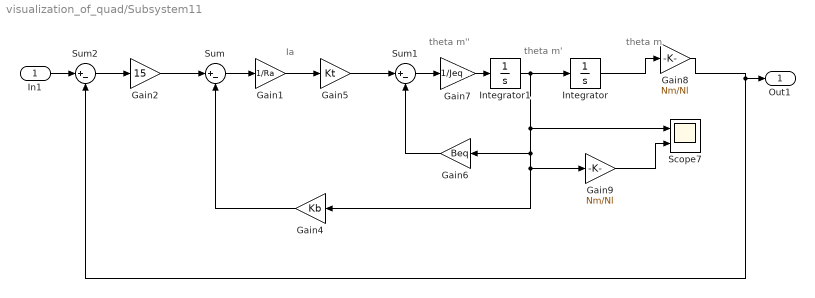
== system visualization_of_quad/Subsystem11 ==
  note: theta m''
  note: theta m'
  note: theta m
  note: Ia
  In1 : Inport
  Gain1 : Gain  Gain=1/Ra
  Gain2 : Gain  Gain=15
  Gain4 : Gain  Gain=Kb
  Gain5 : Gain  Gain=Kt
  Gain6 : Gain  Gain=Beq
  Gain7 : Gain  Gain=1/Jeq
  Gain8 : Gain  Gain=Nm/Nl
  Gain9 : Gain  Gain=Nm/Nl
  Integrator : Integrator
  Integrator1 : Integrator
  Scope7 : Scope  NumInputPorts=2
      settings: YMin=5.04527e-12~1.26132e-12  YMax=5.04527e-12~1.26132e-12  SaveName=ScopeData7
  Sum : Sum  Inputs=|+-
  Sum1 : Sum  Inputs=|+-
  Sum2 : Sum  Inputs=|+-
  Out1 : Outport
  wires:
  Sum/1 -> Gain1/1
  Gain4/1 -> Sum/2
  Integrator1/1 -> Gain9/1, Gain4/1, Gain6/1, Scope7/1, Integrator/1
  Gain1/1 -> Gain5/1
  Gain5/1 -> Sum1/1
  Gain6/1 -> Sum1/2
  Sum1/1 -> Gain7/1
  Gain7/1 -> Integrator1/1
  Integrator/1 -> Gain8/1
  Gain8/1 -> Sum2/2, Out1/1
  Gain9/1 -> Scope7/2
  Sum2/1 -> Gain2/1
  In1/1 -> Sum2/1
  Gain2/1 -> Sum/1

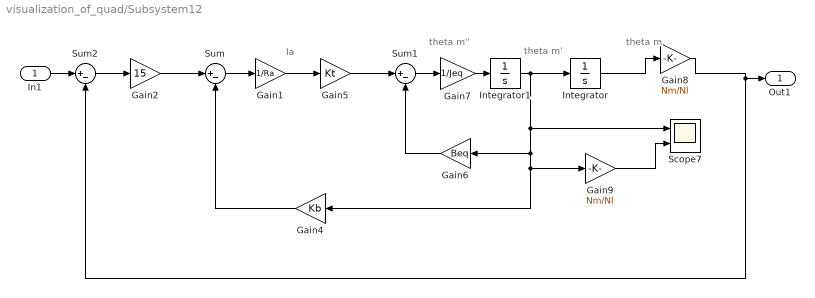
== system visualization_of_quad/Subsystem12 ==
  note: theta m''
  note: theta m'
  note: theta m
  note: Ia
  In1 : Inport
  Gain1 : Gain  Gain=1/Ra
  Gain2 : Gain  Gain=15
  Gain4 : Gain  Gain=Kb
  Gain5 : Gain  Gain=Kt
  Gain6 : Gain  Gain=Beq
  Gain7 : Gain  Gain=1/Jeq
  Gain8 : Gain  Gain=Nm/Nl
  Gain9 : Gain  Gain=Nm/Nl
  Integrator : Integrator
  Integrator1 : Integrator
  Scope7 : Scope  NumInputPorts=2
      settings: YMin=5.04527e-12~1.26132e-12  YMax=5.04527e-12~1.26132e-12  SaveName=ScopeData7
  Sum : Sum  Inputs=|+-
  Sum1 : Sum  Inputs=|+-
  Sum2 : Sum  Inputs=|+-
  Out1 : Outport
  wires:
  Sum/1 -> Gain1/1
  Gain4/1 -> Sum/2
  Integrator1/1 -> Gain9/1, Gain4/1, Gain6/1, Scope7/1, Integrator/1
  Gain1/1 -> Gain5/1
  Gain5/1 -> Sum1/1
  Gain6/1 -> Sum1/2
  Sum1/1 -> Gain7/1
  Gain7/1 -> Integrator1/1
  Integrator/1 -> Gain8/1
  Gain8/1 -> Sum2/2, Out1/1
  Gain9/1 -> Scope7/2
  Sum2/1 -> Gain2/1
  In1/1 -> Sum2/1
  Gain2/1 -> Sum/1

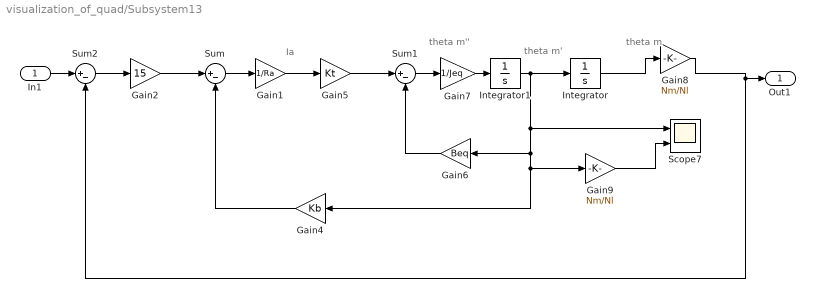
== system visualization_of_quad/Subsystem13 ==
  note: theta m''
  note: theta m'
  note: theta m
  note: Ia
  In1 : Inport
  Gain1 : Gain  Gain=1/Ra
  Gain2 : Gain  Gain=15
  Gain4 : Gain  Gain=Kb
  Gain5 : Gain  Gain=Kt
  Gain6 : Gain  Gain=Beq
  Gain7 : Gain  Gain=1/Jeq
  Gain8 : Gain  Gain=Nm/Nl
  Gain9 : Gain  Gain=Nm/Nl
  Integrator : Integrator
  Integrator1 : Integrator
  Scope7 : Scope  NumInputPorts=2
      settings: YMin=5.04527e-12~1.26132e-12  YMax=5.04527e-12~1.26132e-12  SaveName=ScopeData7
  Sum : Sum  Inputs=|+-
  Sum1 : Sum  Inputs=|+-
  Sum2 : Sum  Inputs=|+-
  Out1 : Outport
  wires:
  Sum/1 -> Gain1/1
  Gain4/1 -> Sum/2
  Integrator1/1 -> Gain9/1, Gain4/1, Gain6/1, Scope7/1, Integrator/1
  Gain1/1 -> Gain5/1
  Gain5/1 -> Sum1/1
  Gain6/1 -> Sum1/2
  Sum1/1 -> Gain7/1
  Gain7/1 -> Integrator1/1
  Integrator/1 -> Gain8/1
  Gain8/1 -> Sum2/2, Out1/1
  Gain9/1 -> Scope7/2
  Sum2/1 -> Gain2/1
  In1/1 -> Sum2/1
  Gain2/1 -> Sum/1

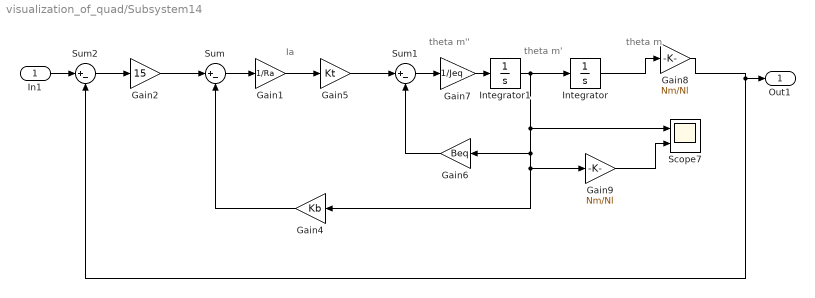
== system visualization_of_quad/Subsystem14 ==
  note: theta m''
  note: theta m'
  note: theta m
  note: Ia
  In1 : Inport
  Gain1 : Gain  Gain=1/Ra
  Gain2 : Gain  Gain=15
  Gain4 : Gain  Gain=Kb
  Gain5 : Gain  Gain=Kt
  Gain6 : Gain  Gain=Beq
  Gain7 : Gain  Gain=1/Jeq
  Gain8 : Gain  Gain=Nm/Nl
  Gain9 : Gain  Gain=Nm/Nl
  Integrator : Integrator
  Integrator1 : Integrator
  Scope7 : Scope  NumInputPorts=2
      settings: YMin=5.04527e-12~1.26132e-12  YMax=5.04527e-12~1.26132e-12  SaveName=ScopeData7
  Sum : Sum  Inputs=|+-
  Sum1 : Sum  Inputs=|+-
  Sum2 : Sum  Inputs=|+-
  Out1 : Outport
  wires:
  Sum/1 -> Gain1/1
  Gain4/1 -> Sum/2
  Integrator1/1 -> Gain9/1, Gain4/1, Gain6/1, Scope7/1, Integrator/1
  Gain1/1 -> Gain5/1
  Gain5/1 -> Sum1/1
  Gain6/1 -> Sum1/2
  Sum1/1 -> Gain7/1
  Gain7/1 -> Integrator1/1
  Integrator/1 -> Gain8/1
  Gain8/1 -> Sum2/2, Out1/1
  Gain9/1 -> Scope7/2
  Sum2/1 -> Gain2/1
  In1/1 -> Sum2/1
  Gain2/1 -> Sum/1

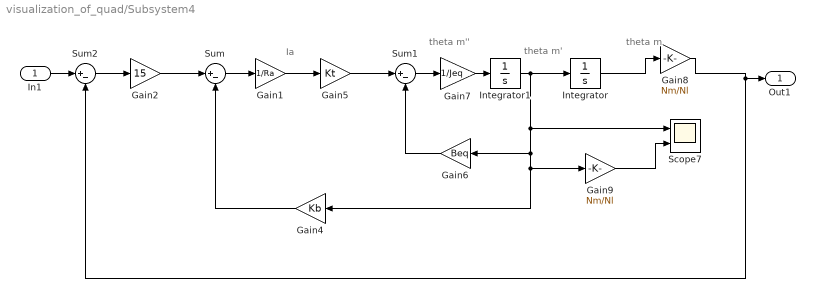
== system visualization_of_quad/Subsystem4 ==
  note: theta m''
  note: theta m'
  note: theta m
  note: Ia
  In1 : Inport
  Gain1 : Gain  Gain=1/Ra
  Gain2 : Gain  Gain=15
  Gain4 : Gain  Gain=Kb
  Gain5 : Gain  Gain=Kt
  Gain6 : Gain  Gain=Beq
  Gain7 : Gain  Gain=1/Jeq
  Gain8 : Gain  Gain=Nm/Nl
  Gain9 : Gain  Gain=Nm/Nl
  Integrator : Integrator
  Integrator1 : Integrator
  Scope7 : Scope  NumInputPorts=2
      settings: YMin=-5~-5  YMax=5~5  SaveName=ScopeData7
  Sum : Sum  Inputs=|+-
  Sum1 : Sum  Inputs=|+-
  Sum2 : Sum  Inputs=|+-
  Out1 : Outport
  wires:
  Sum/1 -> Gain1/1
  Gain4/1 -> Sum/2
  Integrator1/1 -> Gain9/1, Gain4/1, Gain6/1, Scope7/1, Integrator/1
  Gain1/1 -> Gain5/1
  Gain5/1 -> Sum1/1
  Gain6/1 -> Sum1/2
  Sum1/1 -> Gain7/1
  Gain7/1 -> Integrator1/1
  Integrator/1 -> Gain8/1
  Gain8/1 -> Sum2/2, Out1/1
  Gain9/1 -> Scope7/2
  Sum2/1 -> Gain2/1
  In1/1 -> Sum2/1
  Gain2/1 -> Sum/1

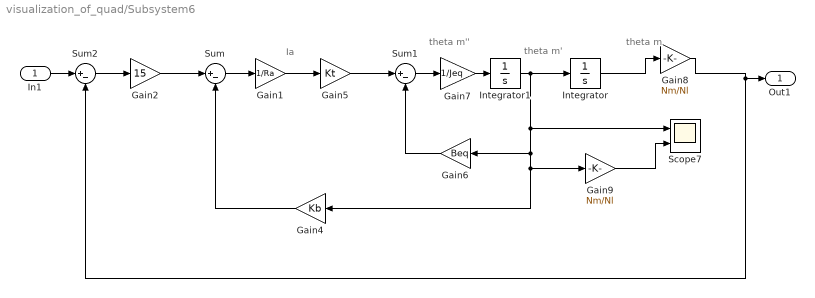
== system visualization_of_quad/Subsystem6 ==
  note: theta m''
  note: theta m'
  note: theta m
  note: Ia
  In1 : Inport
  Gain1 : Gain  Gain=1/Ra
  Gain2 : Gain  Gain=15
  Gain4 : Gain  Gain=Kb
  Gain5 : Gain  Gain=Kt
  Gain6 : Gain  Gain=Beq
  Gain7 : Gain  Gain=1/Jeq
  Gain8 : Gain  Gain=Nm/Nl
  Gain9 : Gain  Gain=Nm/Nl
  Integrator : Integrator
  Integrator1 : Integrator
  Scope7 : Scope  NumInputPorts=2
      settings: YMin=4000~8000  YMax=4000~8000  SaveName=ScopeData7
  Sum : Sum  Inputs=|+-
  Sum1 : Sum  Inputs=|+-
  Sum2 : Sum  Inputs=|+-
  Out1 : Outport
  wires:
  Sum/1 -> Gain1/1
  Gain4/1 -> Sum/2
  Integrator1/1 -> Gain9/1, Gain4/1, Gain6/1, Scope7/1, Integrator/1
  Gain1/1 -> Gain5/1
  Gain5/1 -> Sum1/1
  Gain6/1 -> Sum1/2
  Sum1/1 -> Gain7/1
  Gain7/1 -> Integrator1/1
  Integrator/1 -> Gain8/1
  Gain8/1 -> Sum2/2, Out1/1
  Gain9/1 -> Scope7/2
  Sum2/1 -> Gain2/1
  In1/1 -> Sum2/1
  Gain2/1 -> Sum/1

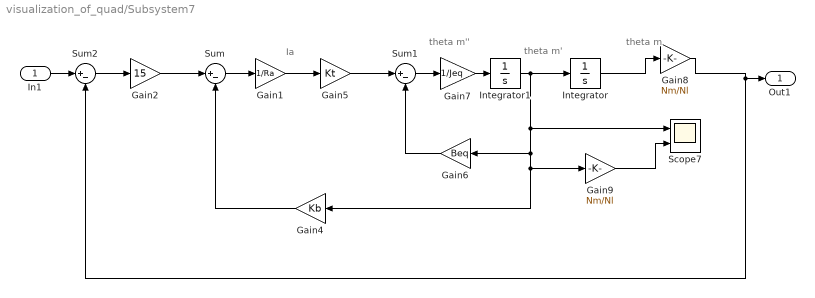
== system visualization_of_quad/Subsystem7 ==
  note: theta m''
  note: theta m'
  note: theta m
  note: Ia
  In1 : Inport
  Gain1 : Gain  Gain=1/Ra
  Gain2 : Gain  Gain=15
  Gain4 : Gain  Gain=Kb
  Gain5 : Gain  Gain=Kt
  Gain6 : Gain  Gain=Beq
  Gain7 : Gain  Gain=1/Jeq
  Gain8 : Gain  Gain=Nm/Nl
  Gain9 : Gain  Gain=Nm/Nl
  Integrator : Integrator
  Integrator1 : Integrator
  Scope7 : Scope  NumInputPorts=2
      settings: YMin=-5~-5  YMax=5~5  SaveName=ScopeData7
  Sum : Sum  Inputs=|+-
  Sum1 : Sum  Inputs=|+-
  Sum2 : Sum  Inputs=|+-
  Out1 : Outport
  wires:
  Sum/1 -> Gain1/1
  Gain4/1 -> Sum/2
  Integrator1/1 -> Gain9/1, Gain4/1, Gain6/1, Scope7/1, Integrator/1
  Gain1/1 -> Gain5/1
  Gain5/1 -> Sum1/1
  Gain6/1 -> Sum1/2
  Sum1/1 -> Gain7/1
  Gain7/1 -> Integrator1/1
  Integrator/1 -> Gain8/1
  Gain8/1 -> Sum2/2, Out1/1
  Gain9/1 -> Scope7/2
  Sum2/1 -> Gain2/1
  In1/1 -> Sum2/1
  Gain2/1 -> Sum/1

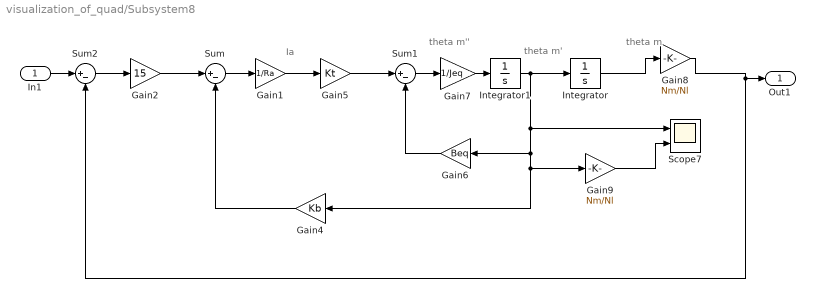
== system visualization_of_quad/Subsystem8 ==
  note: theta m''
  note: theta m'
  note: theta m
  note: Ia
  In1 : Inport
  Gain1 : Gain  Gain=1/Ra
  Gain2 : Gain  Gain=15
  Gain4 : Gain  Gain=Kb
  Gain5 : Gain  Gain=Kt
  Gain6 : Gain  Gain=Beq
  Gain7 : Gain  Gain=1/Jeq
  Gain8 : Gain  Gain=Nm/Nl
  Gain9 : Gain  Gain=Nm/Nl
  Integrator : Integrator
  Integrator1 : Integrator
  Scope7 : Scope  NumInputPorts=2
      settings: YMin=-5~-5  YMax=5~5  SaveName=ScopeData7
  Sum : Sum  Inputs=|+-
  Sum1 : Sum  Inputs=|+-
  Sum2 : Sum  Inputs=|+-
  Out1 : Outport
  wires:
  Sum/1 -> Gain1/1
  Gain4/1 -> Sum/2
  Integrator1/1 -> Gain9/1, Gain4/1, Gain6/1, Scope7/1, Integrator/1
  Gain1/1 -> Gain5/1
  Gain5/1 -> Sum1/1
  Gain6/1 -> Sum1/2
  Sum1/1 -> Gain7/1
  Gain7/1 -> Integrator1/1
  Integrator/1 -> Gain8/1
  Gain8/1 -> Sum2/2, Out1/1
  Gain9/1 -> Scope7/2
  Sum2/1 -> Gain2/1
  In1/1 -> Sum2/1
  Gain2/1 -> Sum/1

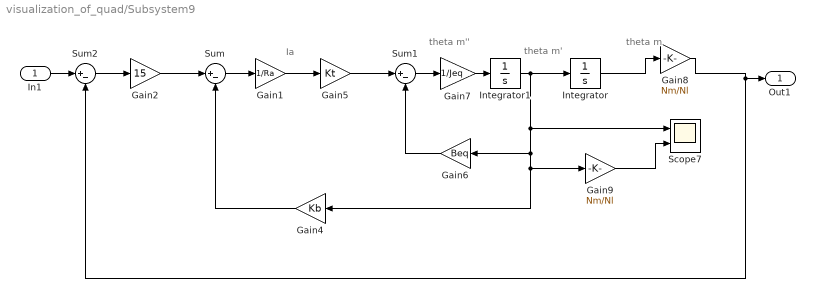
== system visualization_of_quad/Subsystem9 ==
  note: theta m''
  note: theta m'
  note: theta m
  note: Ia
  In1 : Inport
  Gain1 : Gain  Gain=1/Ra
  Gain2 : Gain  Gain=15
  Gain4 : Gain  Gain=Kb
  Gain5 : Gain  Gain=Kt
  Gain6 : Gain  Gain=Beq
  Gain7 : Gain  Gain=1/Jeq
  Gain8 : Gain  Gain=Nm/Nl
  Gain9 : Gain  Gain=Nm/Nl
  Integrator : Integrator
  Integrator1 : Integrator
  Scope7 : Scope  NumInputPorts=2
      settings: YMin=5.04527e-12~1.26132e-12  YMax=5.04527e-12~1.26132e-12  SaveName=ScopeData7
  Sum : Sum  Inputs=|+-
  Sum1 : Sum  Inputs=|+-
  Sum2 : Sum  Inputs=|+-
  Out1 : Outport
  wires:
  Sum/1 -> Gain1/1
  Gain4/1 -> Sum/2
  Integrator1/1 -> Gain9/1, Gain4/1, Gain6/1, Scope7/1, Integrator/1
  Gain1/1 -> Gain5/1
  Gain5/1 -> Sum1/1
  Gain6/1 -> Sum1/2
  Sum1/1 -> Gain7/1
  Gain7/1 -> Integrator1/1
  Integrator/1 -> Gain8/1
  Gain8/1 -> Sum2/2, Out1/1
  Gain9/1 -> Scope7/2
  Sum2/1 -> Gain2/1
  In1/1 -> Sum2/1
  Gain2/1 -> Sum/1

== matlab function visualization_of_quad/MATLAB Function ==
  data: x output; t input; y output; z output
function [x,y,z] = fcn(t)
%#codegen
%t=0:0.2:30*pi;
A=5;a=5;
B=10;b=4;
C=8;c=5;
x=A*cos(a*0.070*t);
y=B*sin(b*0.07*t);
z=C*(1-exp(-5*0.070*t));
%plot3(x,y,z,'r')
%grid on
